simulink model "SOCjisuanmokuai"  (R2015b)
settings: Solver=VariableStepAuto  SolverMode=SingleTasking  StartTime=0.0  StopTime=50  RelTol=1e-3
undefined symbols (not defined in the file): sigbuilder_block
settings Model: Creator=guowe  LastModifiedBy=guowe
settings DataIOCC: LimitDataPoints=off  ReturnWorkspaceOutputs=on
settings DebuggingCC: UnconnectedInputMsg=none  UnconnectedOutputMsg=none  UnconnectedLineMsg=none  AllowSymbolicDim=on  SFUnexpectedBacktrackingDiag=error  SFNoUnconditionalDefaultTransitionDiag=error
settings ModelReferenceCC: EnableRefExpFcnMdlSchedulingChecks=off  PropagateSignalLabelsOutOfModel=on
settings SFSimCC: SimUseLocalCustomCode=on
settings RTWCC: RTWUseLocalCustomCode=on
settings GRTTargetCC: TargetLangStandard=C99 (ISO)
settings ConfigComp: CovMetricSettings=dwe  CovSaveCumulativeToWorkspaceVar=off  CovSaveSingleToWorkspaceVar=off  CovModelRefEnable=Off  CovExternalEMLEnable=on

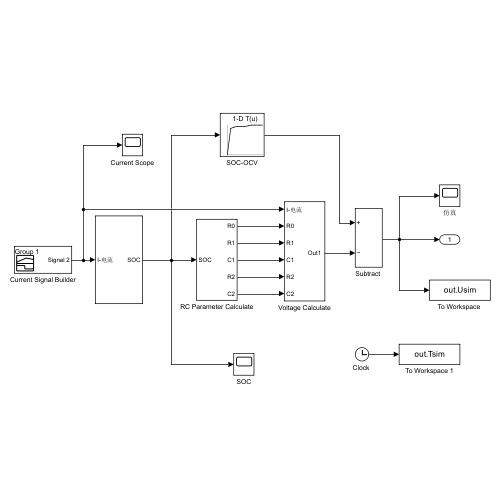
[thumbnail: Simulink's stored preview of the top-level diagram]
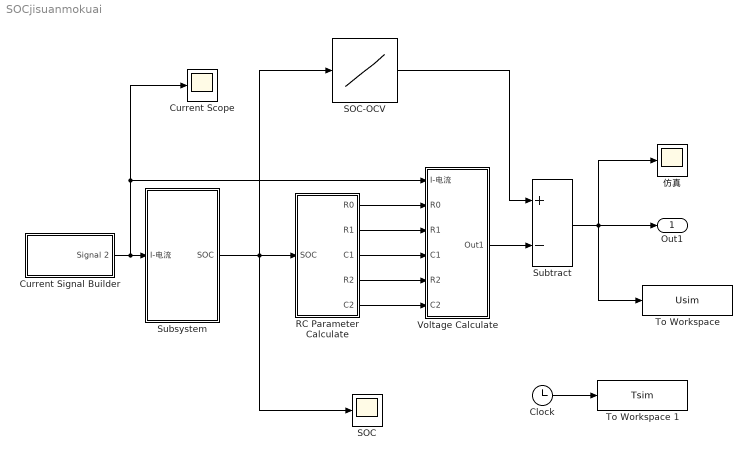
== system SOCjisuanmokuai ==
  "Clock " : Clock
      settings: Decimation=50
  Current Scope : Scope
  Current Signal Builder : Subsystem  Tag=STV Subsys  LoadFcn=sigbuilder_block('load');  StartFcn=sigbuilder_block('start');  StopFcn=sigbuilder_block('stop');  ClipboardFcn=sigbuilder_block('clipboard');  mask(Sigbuilder block){}
      mask help: Simulink:masks:SigbuilderBlock_MD
      mask init:
      | if ~strcmp(get_param(bdroot(gcbh),'SimulationStatus'),'stopped') tuvar = sigbuilder_block('maskInit'); end
      settings: CopyFcn=sigbuilder_block('copy');  DeleteFcn=sigbuilder_block('delete');  ModelCloseFcn=sigbuilder_block('modelClose');  PreSaveFcn=sigbuilder_block('preSave');  PauseFcn=sigbuilder_block('pause');  ContinueFcn=sigbuilder_block('continue');  NameChangeFcn=sigbuilder_block('namechange');  OpenFcn=sigbuilder_block('open',[5.5 36 949 413 ]);  CloseFcn=sigbuilder_block('close');
      mask Display: plot(0, 0, 100, 100,[2, 2, 32, 32, 2], [68, 8, 8, 68, 68],[32, 2], [38, 38], [32, 19, 2],[53, 60, 44], [32, 17, 17, 2],[16, 16, 31, 31]);txt = getActiveGroup(gcbh);text(2, 100, txt,'verticalAlignment', 'top');
  RC Parameter Calculate : Subsystem
  SOC : Scope
  SOC-OCV : Lookup_n-D  NumberOfTableDimensions=1  BreakpointsForDimension1=[0.0 0.1 0.2 0.3 0.4 0.5 0.6 0.7 0.8 0.9 1]  Table=[2.237 3.230 3.277 3.311 3.314 3.316 3.322 3.349 3.350 3.351 3.368]  InternalRulePriority=Speed  RndMeth=Simplest  InputSameDT=on
  Subsystem : Subsystem
  "Subtract " : Sum  Inputs=+-
  "To Workspace " : ToWorkspace  VariableName=Usim  SaveFormat=Timeseries  SampleTime=-1
  To Workspace 1 : ToWorkspace  VariableName=Tsim  SaveFormat=Timeseries  SampleTime=-1
  Voltage Calculate : Subsystem
  仿真 : Scope
  Out1 : Outport
  wires:
  Current Signal Builder/1(Signal 2) -> Current Scope/1, Voltage Calculate/1(I-电流), Subsystem/1(I-电流)
  RC Parameter Calculate/1(R0) -> Voltage Calculate/2(R0)
  RC Parameter Calculate/2(R1) -> Voltage Calculate/3(R1)
  RC Parameter Calculate/3(C1) -> Voltage Calculate/4(C1)
  RC Parameter Calculate/4(R2) -> Voltage Calculate/5(R2)
  RC Parameter Calculate/5(C2) -> Voltage Calculate/6(C2)
  Voltage Calculate/1("Out1 ") -> "Subtract "/2
  SOC-OCV/1 -> "Subtract "/1
  Subsystem/1(SOC) -> RC Parameter Calculate/1(SOC), SOC/1, SOC-OCV/1
  "Subtract "/1 -> "To Workspace "/1, 仿真/1, Out1/1
  "Clock "/1 -> To Workspace 1/1

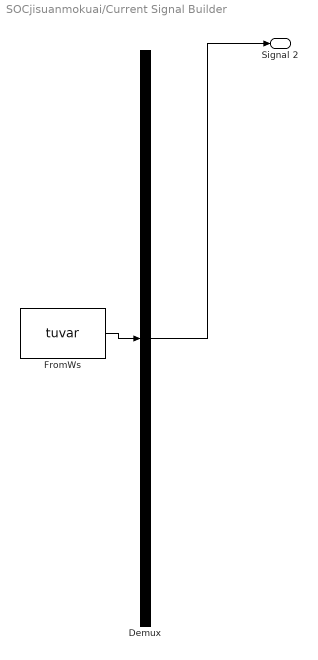
== system SOCjisuanmokuai/Current Signal Builder ==
  Demux : Demux  Tag=STV Demux  Outputs=1
      settings: DisplayOption=none
  FromWs : FromWorkspace  Tag=STV FromWs  VariableName=tuvar
      SigBuilderData=|
      | common.afterFinalStr = 'Extrapolate'
      | common.sampleTime = 0
      | dataSet.timeRange = [0 50]
      | dataSet.name = 'Group 1'
      | sbobj.Groups.Name = 'Group 1'
      | sbobj.Groups.Signals.Name = 'Signal 2'
      | sbobj.Groups.Signals.XData = [0 10.05 10.25 50]
      | sbobj.Groups.Signals.YData = [1.35 1.35 0 0]
      | sbobj.Groups.TimeRange = [0 50]
  Signal 2 : Outport  Tag=STV Outport
  wires:
  FromWs/1 -> Demux/1
  Demux/1 -> Signal 2/1

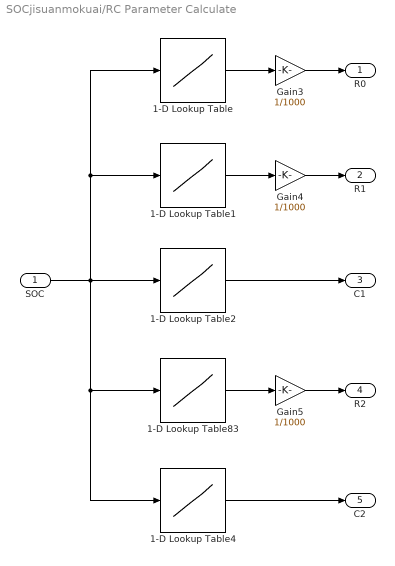
== system SOCjisuanmokuai/RC Parameter Calculate ==
  SOC : Inport
  "1-D Lookup Table " : Lookup_n-D  NumberOfTableDimensions=1  BreakpointsForDimension1=[0.1 0.2 0.3 0.4 0.5 0.6 0.7 0.8 0.9]  Table=[92.037 92.5925 90 84.074 80.37 79.2595 78.5185 75.5555 74.074]  InternalRulePriority=Speed  RndMeth=Simplest  InputSameDT=on
  "1-D Lookup Table1 " : Lookup_n-D  NumberOfTableDimensions=1  BreakpointsForDimension1=[0.1 0.2 0.3 0.4 0.5 0.6 0.7 0.8 0.9]  Table=[32.444 10.800 8.407 6.647 7.496 7.919 7.859 4.832 7.096]  InternalRulePriority=Speed  RndMeth=Simplest  InputSameDT=on
  "1-D Lookup Table2 " : Lookup_n-D  NumberOfTableDimensions=1  BreakpointsForDimension1=[0.1 0.2 0.3 0.4 0.5 0.6 0.7 0.8 0.9]  Table=[54.960 121.674 146.389 425.919 229.409 195.097 443.340 277.612 167.920]  InternalRulePriority=Speed  RndMeth=Simplest  InputSameDT=on
  "1-D Lookup Table4 " : Lookup_n-D  NumberOfTableDimensions=1  BreakpointsForDimension1=[0.1 0.2 0.3 0.4 0.5 0.6 0.7 0.8 0.9]  Table=[498.253 1532.990 2513.583 1619.937 1471.419 1530.717 2878.646 1217.499 1672.882]  InternalRulePriority=Speed  RndMeth=Simplest  InputSameDT=on
  "1-D Lookup Table83 " : Lookup_n-D  NumberOfTableDimensions=1  BreakpointsForDimension1=[0.1 0.2 0.3 0.4 0.5 0.6 0.7 0.8 0.9]  Table=[29.370 18.481 15.511 12.504 13.156 11.585 12.852 13.430 10.837]  InternalRulePriority=Speed  RndMeth=Simplest  InputSameDT=on
  Gain3 : Gain  Gain=1/1000
  Gain4 : Gain  Gain=1/1000
  Gain5 : Gain  Gain=1/1000
  R0 : Outport
  R1 : Outport  Port=2
  C1 : Outport  Port=3
  R2 : Outport  Port=4
  C2 : Outport  Port=5
  wires:
  Gain5/1 -> R2/1
  "1-D Lookup Table2 "/1 -> C1/1
  "1-D Lookup Table "/1 -> Gain3/1
  SOC/1 -> "1-D Lookup Table2 "/1, "1-D Lookup Table "/1, "1-D Lookup Table1 "/1, "1-D Lookup Table4 "/1, "1-D Lookup Table83 "/1
  "1-D Lookup Table4 "/1 -> C2/1
  "1-D Lookup Table1 "/1 -> Gain4/1
  "1-D Lookup Table83 "/1 -> Gain5/1
  Gain4/1 -> R1/1
  Gain3/1 -> R0/1

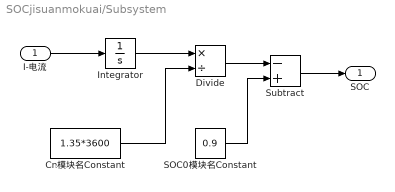
== system SOCjisuanmokuai/Subsystem ==
  I-电流 : Inport
  Cn模块名Constant : Constant  Value=1.35*3600
  "Divide " : Product  Inputs=*/
  "Integrator " : Integrator
  SOC0模块名Constant : Constant  Value=0.9
  "Subtract " : Sum  Inputs=-+
  SOC : Outport
  wires:
  "Divide "/1 -> "Subtract "/1
  Cn模块名Constant/1 -> "Divide "/2
  SOC0模块名Constant/1 -> "Subtract "/2
  "Integrator "/1 -> "Divide "/1
  I-电流/1 -> "Integrator "/1
  "Subtract "/1 -> SOC/1

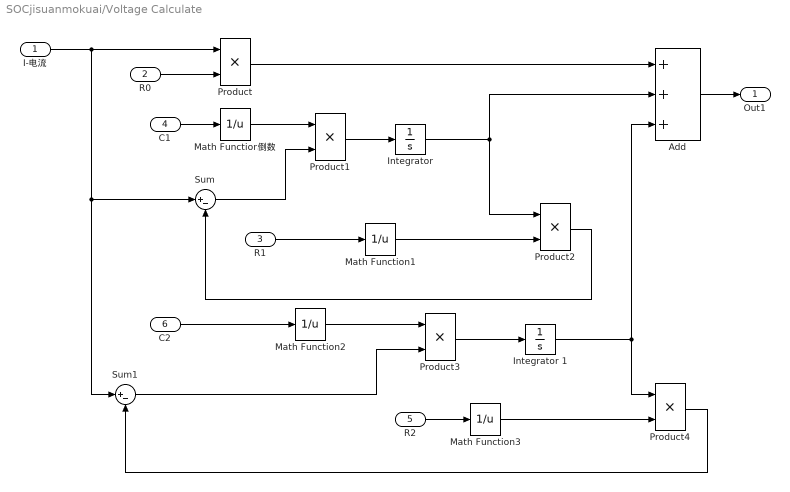
== system SOCjisuanmokuai/Voltage Calculate ==
  I-电流 : Inport
  R0 : Inport  Port=2
  R1 : Inport  Port=3
  C1 : Inport  Port=4
  R2 : Inport  Port=5
  C2 : Inport  Port=6
  "Add " : Sum  Inputs=+++
  "Integrator " : Integrator
  Integrator 1 : Integrator
  "Math Function1 " : Math  Operator=reciprocal  SaturateOnIntegerOverflow=on
  "Math Function2 " : Math  Operator=reciprocal  SaturateOnIntegerOverflow=on
  "Math Function3 " : Math  Operator=reciprocal  SaturateOnIntegerOverflow=on
  Math Function倒数 : Math  Operator=reciprocal  SaturateOnIntegerOverflow=on
  "Product " : Product
  "Product1 " : Product
  "Product2 " : Product
  "Product3 " : Product
  "Product4 " : Product
  Sum : Sum  Inputs=|+-
  Sum1 : Sum  Inputs=|+-
  "Out1 " : Outport
  wires:
  "Add "/1 -> "Out1 "/1
  Math Function倒数/1 -> "Product1 "/1
  "Integrator "/1 -> "Product2 "/1, "Add "/2
  R2/1 -> "Math Function3 "/1
  "Product "/1 -> "Add "/1
  "Math Function1 "/1 -> "Product2 "/2
  C2/1 -> "Math Function2 "/1
  "Product1 "/1 -> "Integrator "/1
  "Product2 "/1 -> Sum/2
  Sum/1 -> "Product1 "/2
  I-电流/1 -> "Product "/1, Sum1/1, Sum/1
  C1/1 -> Math Function倒数/1
  Sum1/1 -> "Product3 "/2
  "Math Function3 "/1 -> "Product4 "/2
  "Math Function2 "/1 -> "Product3 "/1
  "Product3 "/1 -> Integrator 1/1
  "Product4 "/1 -> Sum1/2
  R0/1 -> "Product "/2
  R1/1 -> "Math Function1 "/1
  Integrator 1/1 -> "Product4 "/1, "Add "/3
